simulink model "TestModel_MultiRate"  (R2012b)
settings: Solver=FixedStepDiscrete  SolverMode=SingleTasking  StartTime=0.0  StopTime=10.0  FixedStep=0.005  RelTol=1e-3
settings Model: BufferReuse=off  Creator=freyjed  LastModifiedBy=freyjed
settings OptimizationCC: BlockReduction=off  ConditionallyExecuteInputs=off  BufferReuse=off  OptimizeModelRefInitCode=on  LifeSpan=1
settings HardwareCC: ProdLargestAtomicInteger=Integer  ProdLargestAtomicFloat=Float  ProdIntDivRoundTo=Zero  ProdEndianess=LittleEndian  ProdHWDeviceType=ChibiOS->ChibiOS  TargetLargestAtomicInteger=Integer  TargetLargestAtomicFloat=Float  TargetIntDivRoundTo=Zero  TargetEndianess=LittleEndian  TargetHWDeviceType=ChibiOS->ChibiOS
settings ModelReferenceCC: UpdateModelReferenceTargets=Force
settings RTWCC: SystemTargetFile=ert.tlc  GenCodeOnly=on  TemplateMakefile=ert_default_tmf  Description=Embedded Coder  ProcessScript=ert_make_rtw_hook
settings CodeAppCC: ForceParamTrailComments=on  IgnoreCustomStorageClasses=off  OperatorAnnotations=on  SimulinkDataObjDesc=on  SFDataObjDesc=on  MATLABFcnDesc=on  DefineNamingRule=UpperCase  InsertBlockDesc=on  MATLABSourceComments=on  ReqsInCode=on
settings ERTTargetCC: CodeReplacementLibrary=C99 (ISO)  MultiwordLength=2048  GenerateSampleERTMain=on  SupportAbsoluteTime=off  SupportComplex=off  SupportNonInlinedSFcns=on  ParenthesesLevel=Maximum  ERTCustomFileTemplate=example_file_process.tlc  PreserveExpressionOrder=on  PreserveIfCondition=on  SuppressUnreachableDefaultCases=off

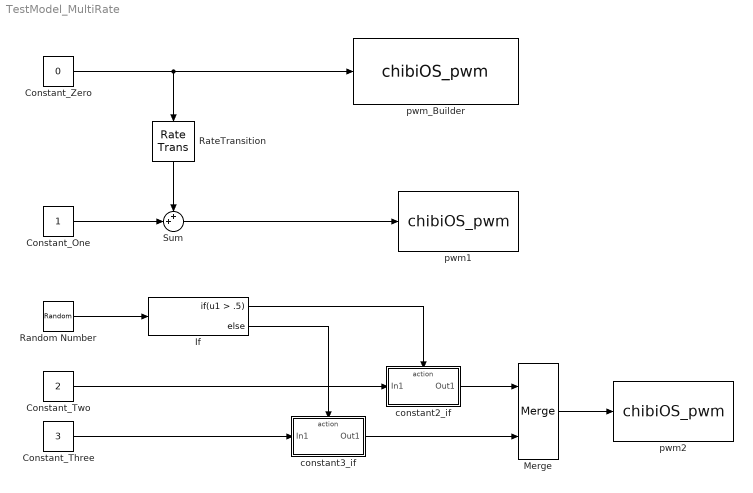
== system TestModel_MultiRate ==
  Constant_One : Constant  OutDataTypeStr=Inherit: Inherit via back propagation  SampleTime=0.015
  Constant_Three : Constant  Value=3  OutDataTypeStr=Inherit: Inherit via back propagation  SampleTime=0.1
  Constant_Two : Constant  Value=2  OutDataTypeStr=Inherit: Inherit via back propagation  SampleTime=0.1
  Constant_Zero : Constant  Value=0  OutDataTypeStr=Inherit: Inherit via back propagation  SampleTime=0.005
  If : If  IfExpression=u1 > .5
  Merge : Merge
  Random Number : RandomNumber  Mean=.5
  RateTransition : RateTransition  OutPortSampleTimeOpt=Inherit
  Sum : Sum  Inputs=++|  SampleTime=0.015
  constant2_if : Subsystem  TreatAsAtomicUnit=on
  constant3_if : Subsystem  TreatAsAtomicUnit=on
  pwm1 : S-Function  FunctionName=chibiOS_pwm  Parameters=int16(clockFrequency),int16(clockPeriod)  EnableBusSupport=off  mask{clockFrequency=2000, clockPeriod=500}
      mask prompts: clockFrequency "Clock Frequency"; clockPeriod "Clock Period"
  pwm2 : S-Function  FunctionName=chibiOS_pwm  Parameters=int16(clockFrequency),int16(clockPeriod)  EnableBusSupport=off  mask{clockFrequency=2000, clockPeriod=500}
      mask prompts: clockFrequency "Clock Frequency"; clockPeriod "Clock Period"
  pwm_Builder : S-Function  InitFcn=try, set_param(gcb,'FunctionName','chibiOS_pwm'), end  FunctionName=chibiOS_pwm  Parameters=int16(10000),int16(10000)  SFunctionModules=chibiOS_pwm_wrapper  EnableBusSupport=off  mask(S-Function Builder){}
      mask help: Simulink:masks:SFunctionBuilder_MD
      mask init:
      | val = [[.9  0.75 0.75 1 1 .9 .9 1]',[1 1 0.75 0.75 .9 .9 1 .9]'];try , sys = get_param(gcb,'SfunBuilderFcnName');if isempty(sys), sys = get_param(gcb,'FunctionName'); end,catch, sys = get_param(gcb,'FunctionName'); end
      settings: CopyFcn=set_param(gcbh,'LinkStatus','none')  PreSaveFcn=try, set_param(gcb,'FunctionName','chibiOS_pwm'), end  OpenFcn=sfunctionwizard(gcbh)
      mask Display: plot(val(:,1),val(:,2)),disp(sys), port_label('input',1,'Input')
  wires:
  Constant_Zero/1 -> RateTransition/1, pwm_Builder/1
  Sum/1 -> pwm1/1
  Constant_One/1 -> Sum/2
  RateTransition/1 -> Sum/1
  Constant_Two/1 -> constant2_if/1(In1)
  Constant_Three/1 -> constant3_if/1(In1)
  constant2_if/1(Out1) -> Merge/1
  constant3_if/1(Out1) -> Merge/2
  Merge/1 -> pwm2/1
  If/2 -> constant3_if/Action
  If/1 -> constant2_if/Action
  Random Number/1 -> If/1

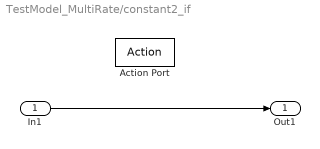
== system TestModel_MultiRate/constant2_if ==
  In1 : Inport
  Action Port : ActionPort  ActionType=then
  Out1 : Outport
  wires:
  In1/1 -> Out1/1

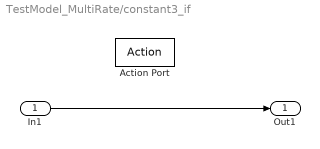
== system TestModel_MultiRate/constant3_if ==
  In1 : Inport
  Action Port : ActionPort  ActionType=else
  Out1 : Outport
  wires:
  In1/1 -> Out1/1
